simulink model "dsp_proj_ram_testing"  (R2025a)
settings: Solver=VariableStepAuto  StartTime=0.0  StopTime=10.0  RelTol=1e-3
libraries: hdlsllib x4, simulink x1
settings Model: Creator=UTSAB KARAN  LastModifiedBy=rs130

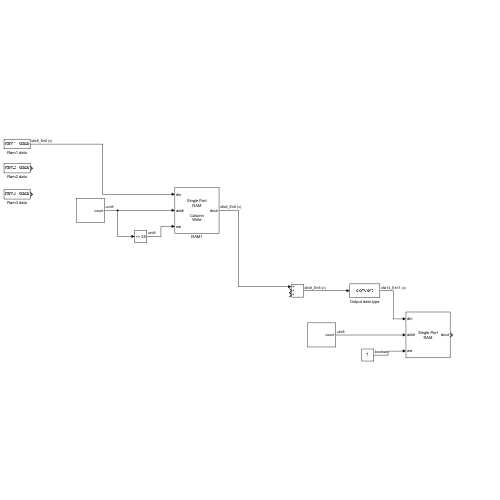
[thumbnail: Simulink's stored preview of the top-level diagram]
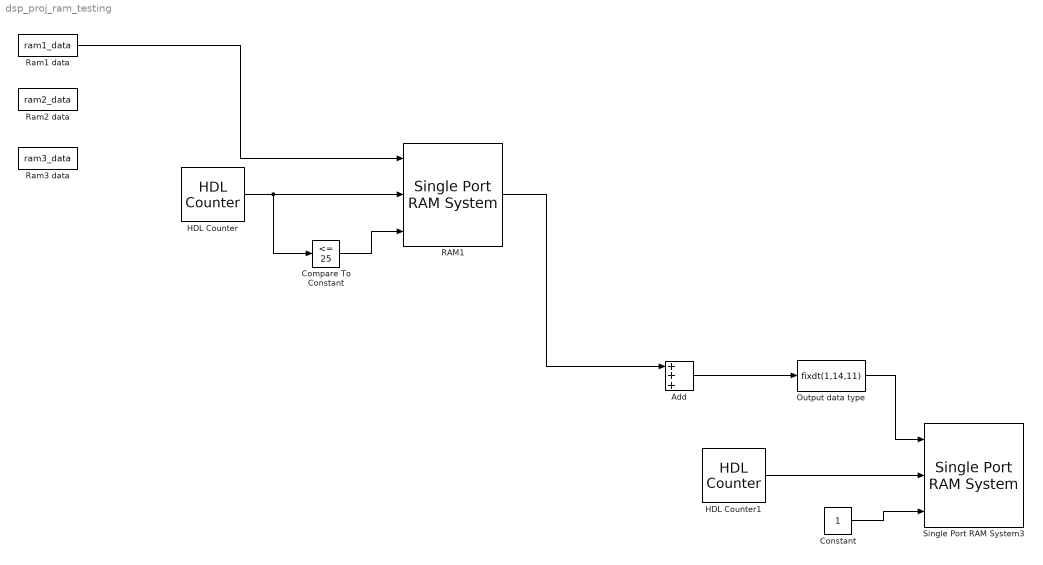
== system dsp_proj_ram_testing ==
  Add : Sum  Inputs=+++
  Compare To Constant : simulink/Logic and Bit Operations/Compare To Constant  relop=<=  const=25  OutDataTypeStr=uint8
  Constant : Constant  OutDataTypeStr=boolean
  HDL Counter : hdlsllib/Sources/HDL Counter  CountType=Count limited  CountInit=0  CountStep=1  CountMax=50  CountFromType=Initial value  CountFrom=0  CountResetPort=off  CountLoadPort=off  CountEnbPort=off  CountDirPort=off  CountHitOutputPort=off  CountDataType=Unsigned  CountWordLen=8  CountFracLen=0  CountSampTime=1
  HDL Counter1 : hdlsllib/Sources/HDL Counter  CountType=Count limited  CountInit=0  CountStep=1  CountMax=50  CountFromType=Initial value  CountFrom=0  CountResetPort=off  CountLoadPort=off  CountEnbPort=off  CountDirPort=off  CountHitOutputPort=off  CountDataType=Unsigned  CountWordLen=8  CountFracLen=0  CountSampTime=1
  Output data type : DataTypeConversion  OutDataTypeStr=fixdt(1,14,11)  SaturateOnIntegerOverflow=off  RndMeth=Floor  LockScale=on
  RAM1 : hdlsllib/HDL RAMs/Single Port RAM System  RAMType=Single port  AsyncRead=off  WriteOutputValue=New data  RAMInitialValue=0  allowBusInputs=off  WritesHaveOutput=on  NumReads=0  NumWrites=1  SimulateUsing=Code generation  ModelRAMDelay=on  VectorAccess=Parallel
  Ram1 data : FromWorkspace  VariableName=ram1_data  Interpolate=off  OutputAfterFinalValue=Holding final value
  Ram2 data : FromWorkspace  VariableName=ram2_data  Interpolate=off  OutputAfterFinalValue=Holding final value
  Ram3 data : FromWorkspace  VariableName=ram3_data  Interpolate=off  OutputAfterFinalValue=Holding final value
  Single Port RAM System3 : hdlsllib/HDL RAMs/Single Port RAM System  RAMType=Single port  AsyncRead=off  WriteOutputValue=New data  RAMInitialValue=0  allowBusInputs=off  WritesHaveOutput=on  NumReads=0  NumWrites=1  SimulateUsing=Code generation  ModelRAMDelay=on  VectorAccess=Parallel
  wires:
  RAM1/1 -> Add/1
  Add/1 -> Output data type/1
  Output data type/1 -> Single Port RAM System3/1
  Ram1 data/1 -> RAM1/1
  HDL Counter/1 -> Compare To Constant/1, RAM1/2
  Compare To Constant/1 -> RAM1/3
  HDL Counter1/1 -> Single Port RAM System3/2
  Constant/1 -> Single Port RAM System3/3
